simulink model "body_acc"  (R2019a)
settings: Solver=FixedStepAuto  StartTime=0.0  StopTime=inf  FixedStep=sT  RelTol=1e-3  EnableMultiTasking=on
InitFcn:
  | clear;
  | init_robot;
  | param;
values from neighbouring files (symbols this model uses):
  g = 9.80665    [param.m]    (also in sim_param.m)
  sT = 0.02    [param.m]    (also in sim_param.m = 0.001)
libraries: raspberrypilib x6, cstblocks x3
settings Model: SimulationMode=external  Creator=hideaki  LastModifiedBy=hideaki
settings SolverCC: PositivePriorityOrder=on
settings OptimizationCC: EnhancedBackFolding=on  PassReuseOutputArgsAs=Individual arguments  MaxStackSize=64  OptimizeBlockOrder=speed  DifferentSizesBufferReuse=on  OptimizationCustomize=off
settings DebuggingCC: ParameterTunabilityLossMsg=error  UnderSpecifiedDimensionMsg=warning
settings HardwareCC: ProdBitPerPointer=32  ProdBitPerSizeT=32  ProdBitPerPtrDiffT=32  ProdLargestAtomicInteger=Long  ProdLargestAtomicFloat=Double  ProdWordSize=32  ProdLongLongMode=on  ProdHWDeviceType=ARM Compatible->ARM Cortex  UseEmbeddedCoderFeatures=off  UseSimulinkCoderFeatures=off
settings SFSimCC: MATLABDynamicMemAlloc=off
settings RTWCC: SystemTargetFile=ert.tlc  HardwareBoard=Raspberry Pi  TLCOptions="-aInlineSetEventsForThisBaseRateFcn=TLC_FALSE -aSuppressMultiTaskScheduler=TLC_FALSE  -aRateBasedStepFcn=0"  TemplateMakefile=ert_default_tmf  RTWVerbose=off  Toolchain=GNU GCC Raspberry Pi  BuildConfiguration=Faster Runs  IncludeHyperlinkInReport=on
settings CodeAppCC: ForceParamTrailComments=on  OperatorAnnotations=on  SimulinkDataObjDesc=on  SFDataObjDesc=on  MangleLength=10  InsertBlockDesc=on
settings ERTTargetCC: SupportNonInlinedSFcns=on  SupportVariableSizeSignals=on  ExtMode=on  ExtModeMexArgs='192.168.10.103' 0 17725  ERTSrcFileBannerTemplate=codertarget_code_template.cgt  ERTHdrFileBannerTemplate=codertarget_code_template.cgt  ERTDataSrcFileTemplate=codertarget_code_template.cgt  ERTDataHdrFileTemplate=codertarget_code_template.cgt

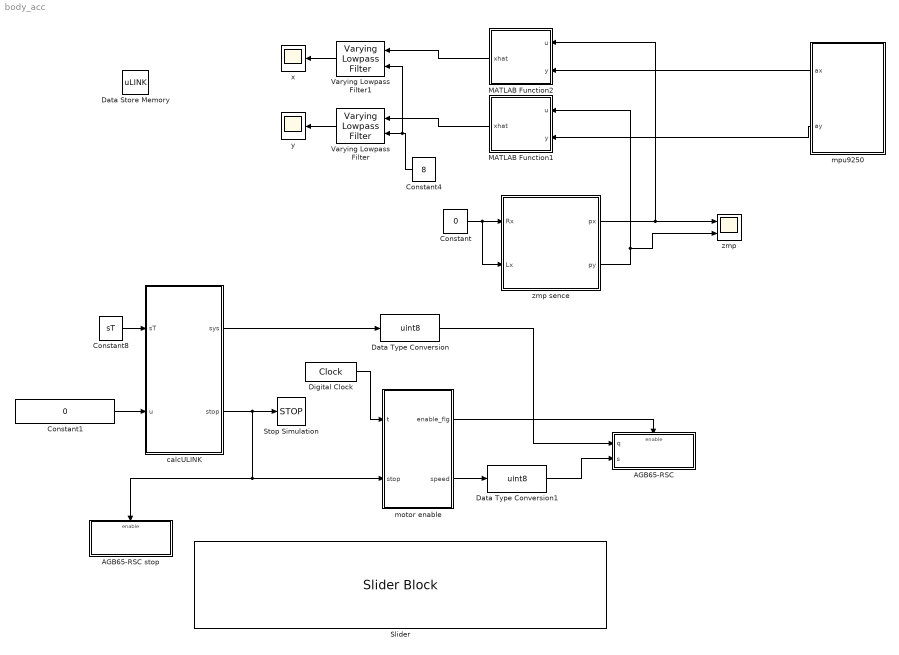
== system body_acc ==
  AGB65-RSC : Subsystem  TreatAsAtomicUnit=on
  AGB65-RSC stop : Subsystem  TreatAsAtomicUnit=on
  Constant : Constant  Value=0
  Constant1 : Constant  Value=0  OutDataTypeStr=double
  Constant4 : Constant  Value=8
  Constant8 : Constant  Value=sT
  Data Store Memory : DataStoreMemory  DataStoreName=uLINK  ReadBeforeWriteMsg=warning  WriteAfterWriteMsg=warning  WriteAfterReadMsg=warning  InitialValue=uLINK  ShowAdditionalParam=off  OutDataTypeStr=Bus: ULINK  Dimensions=[15 1]
  Data Type Conversion : DataTypeConversion  OutDataTypeStr=uint8
  Data Type Conversion1 : DataTypeConversion  OutDataTypeStr=uint8
  Digital Clock : DigitalClock  SampleTime=sT
  MATLAB Function1 : MATLAB Function  TreatAsAtomicUnit=on
  MATLAB Function2 : MATLAB Function  TreatAsAtomicUnit=on
  Slider : SliderBlock  LabelPosition=Hide  ScaleMin=-0.050000000000000003  ScaleMax=0.050000000000000003
  Stop Simulation : Stop
  Varying Lowpass Filter : cstblocks/Linear Parameter Varying/Varying Lowpass Filter  N=1
      settings: SourceProductName=Control System Toolbox
  Varying Lowpass Filter1 : cstblocks/Linear Parameter Varying/Varying Lowpass Filter  N=1
      settings: SourceProductName=Control System Toolbox
  calcULINK : MATLAB Function  TreatAsAtomicUnit=on
  motor enable : MATLAB Function  TreatAsAtomicUnit=on
  mpu9250 : Subsystem
  x : Scope
  y : Scope
  zmp : Scope  NumInputPorts=2
  zmp sence : Subsystem
  wires:
  Constant8/1 -> calcULINK/1(sT)
  Digital Clock/1 -> motor enable/1(t)
  Data Type Conversion1/1 -> AGB65-RSC/2(s)
  motor enable/1(enable_flg) -> AGB65-RSC/Enable
  Data Type Conversion/1 -> AGB65-RSC/1(q)
  calcULINK/1(sys) -> Data Type Conversion/1
  motor enable/2(speed) -> Data Type Conversion1/1
  calcULINK/2(stop) -> AGB65-RSC stop/Enable, motor enable/2(stop), Stop Simulation/1
  Constant/1 -> zmp sence/2(Lx), zmp sence/1(Rx)
  zmp sence/1(px) -> MATLAB Function2/1(u), zmp/1
  zmp sence/2(py) -> MATLAB Function1/1(u), zmp/2
  mpu9250/1(ax) -> MATLAB Function2/2(y)
  mpu9250/2(ay) -> MATLAB Function1/2(y)
  MATLAB Function1/1(xhat) -> Varying Lowpass Filter/1
  MATLAB Function2/1(xhat) -> Varying Lowpass Filter1/1
  Constant1/1 -> calcULINK/2(u)
  Constant4/1 -> Varying Lowpass Filter1/2, Varying Lowpass Filter/2
  Varying Lowpass Filter/1 -> y/1
  Varying Lowpass Filter1/1 -> x/1

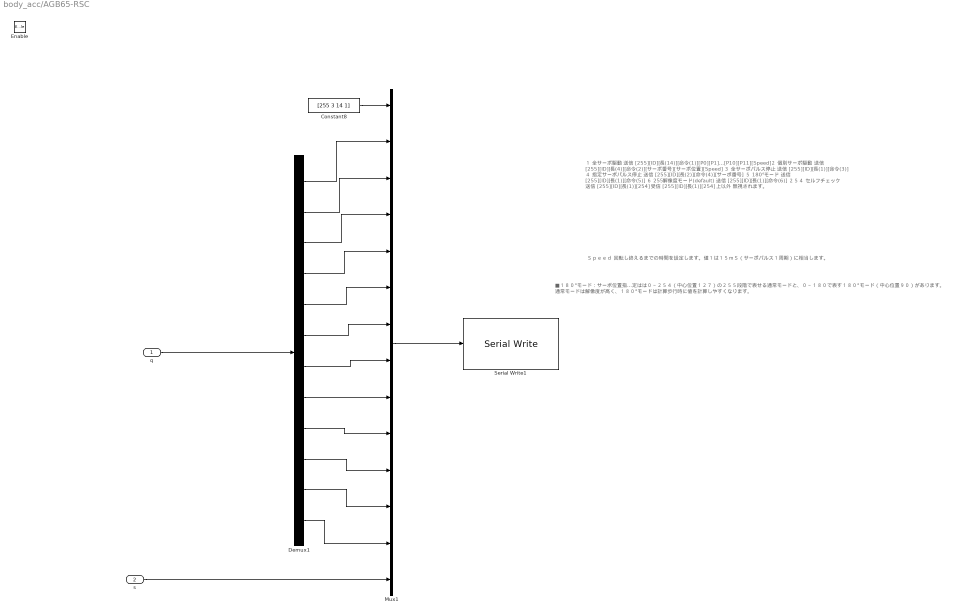
== system body_acc/AGB65-RSC ==
  note: Ｓｐｅｅｄ 回転し終えるまでの時間を設定します。値１は１５ｍＳ（サーボパルス１周期）に相当します。
  note: １ 全サーボ駆動 送信 [255][ID][長(14)][命令(1)][P0][P1]...[P10][P11][Speed]
      | ２ 個別サーボ駆動 送信 [255][ID][長(4)][命令(2)][サーボ番号][サーボ位置][Speed]
      | ３ 全サーボパルス停止 送信 [255][ID][長(1)][命令(3)]
      | ４ 指定サーボパルス停止 送信 [255][ID][長(2)][命令(4)][サーボ番号]
      | ５ 180°モード 送信 [255][ID][長(1)][命令(5)]
      | ６ 255解像度モード(default) 送信 [255][ID][長(1)][命令(6)]
      | ２５４ セルフチェック 送信 [255][ID][長(1)][254] 受信 [255][ID][長(1)][254]
      | 上以外 無視されます。
  note: ■１８０°モード：サーボ位置指定はは０～２５４（中心位置１２７）の２５５段階で表せる通常モードと、０～１８０で表す１８０°モード（中心位置９０）があります。
      | 通常モードは解像度が高く、１８０°モードは計算歩行時に値を計算しやすくなります。
  q : Inport
  s : Inport  Port=2
  Enable : EnablePort
  Constant8 : Constant  Value=[255 3 14 1]  OutDataTypeStr=uint8
  Demux1 : Demux  Outputs=12
  Mux1 : Mux  Inputs=14
  Serial Write1 : raspberrypilib/Serial Write  Priority=1  board=Pi 3 Model B  SCIModule_=/dev/ttyS0  Baudrate_=115200  Parity=None  StopBits_=1  HardwareFlowControl=None  ByteOrder=LittleEndian  OutputStatus=off  blockPlatform=RaspberryPi
      settings: SourceProductName=Simulink Support Package for Raspberry Pi Hardware  SourceProductBaseCode=RASPPI
  wires:
  Constant8/1 -> Mux1/1
  Demux1/11 -> Mux1/12
  q/1 -> Demux1/1
  Demux1/1 -> Mux1/2
  Demux1/3 -> Mux1/4
  Demux1/2 -> Mux1/3
  Mux1/1 -> Serial Write1/1
  Demux1/6 -> Mux1/7
  Demux1/10 -> Mux1/11
  Demux1/5 -> Mux1/6
  Demux1/7 -> Mux1/8
  Demux1/8 -> Mux1/9
  s/1 -> Mux1/14
  Demux1/9 -> Mux1/10
  Demux1/12 -> Mux1/13
  Demux1/4 -> Mux1/5

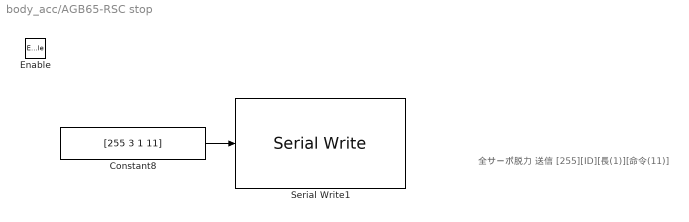
== system body_acc/AGB65-RSC stop ==
  note: 全サーボ脱力 送信 [255][ID][長(1)][命令(11)]
  Enable : EnablePort
  Constant8 : Constant  Value=[255 3 1 11]  OutDataTypeStr=uint8
  Serial Write1 : raspberrypilib/Serial Write  Priority=1  board=Pi 3 Model B  SCIModule_=/dev/ttyS0  Baudrate_=115200  Parity=None  StopBits_=1  HardwareFlowControl=None  ByteOrder=LittleEndian  OutputStatus=off  blockPlatform=RaspberryPi
      settings: SourceProductName=Simulink Support Package for Raspberry Pi Hardware  SourceProductBaseCode=RASPPI
  wires:
  Constant8/1 -> Serial Write1/1

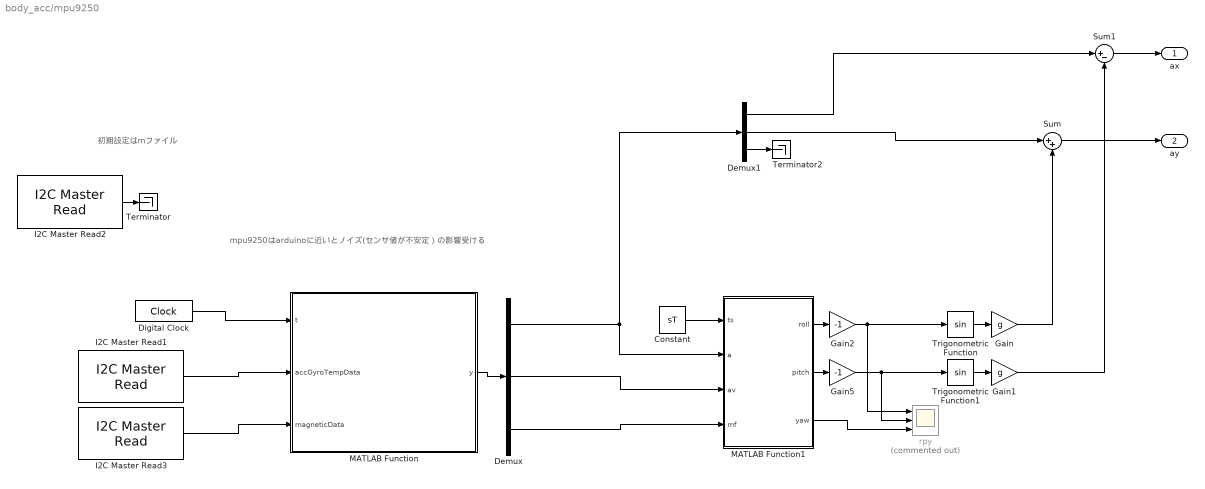
== system body_acc/mpu9250 ==
  note: mpu9250はarduinoに近いとノイズ(センサ値が不安定）の影響受ける
  note: 初期設定はmファイル
  Constant : Constant  Value=sT
  Demux : Demux  Outputs=3
  Demux1 : Demux  Outputs=3
  Digital Clock : DigitalClock  SampleTime=sT
  Gain : Gain  Gain=g
  Gain1 : Gain  Gain=g
  Gain2 : Gain  Gain=-1
  Gain5 : Gain  Gain=-1
  I2C Master Read1 : raspberrypilib/I2C Master Read  BoardProperty=Pi 3 Model B  Mode=Master  SlaveAddress=hex2dec( '68' )  SlaveByteOrder=BigEndian  Direction=Receiver  RegisterAddressMode=on  RegisterAddress=hex2dec( '3b' )  SlaveDataType=uint8  DataLength=14  NoAck=off  RepeatedStart=off  OutputStatus=off  SampleTime=-1
      settings: SourceProductName=Simulink Support Package for Raspberry Pi Hardware  SourceProductBaseCode=RASPPI
  I2C Master Read2 : raspberrypilib/I2C Master Read  BoardProperty=Pi 3 Model B  Mode=Master  SlaveAddress=hex2dec( '0c' )  SlaveByteOrder=BigEndian  Direction=Receiver  RegisterAddressMode=on  RegisterAddress=hex2dec( '02' )  SlaveDataType=uint8  DataLength=1  NoAck=off  RepeatedStart=off  OutputStatus=off  SampleTime=-1
      settings: SourceProductName=Simulink Support Package for Raspberry Pi Hardware  SourceProductBaseCode=RASPPI
  I2C Master Read3 : raspberrypilib/I2C Master Read  BoardProperty=Pi 3 Model B  Mode=Master  SlaveAddress=hex2dec( '0c' )  SlaveByteOrder=BigEndian  Direction=Receiver  RegisterAddressMode=on  RegisterAddress=hex2dec( '03' )  SlaveDataType=uint8  DataLength=7  NoAck=off  RepeatedStart=off  OutputStatus=off  SampleTime=-1
      settings: SourceProductName=Simulink Support Package for Raspberry Pi Hardware  SourceProductBaseCode=RASPPI
  MATLAB Function : MATLAB Function  TreatAsAtomicUnit=on
  MATLAB Function1 : MATLAB Function  TreatAsAtomicUnit=on
  Sum : Sum  Inputs=|++
  Sum1 : Sum  Inputs=|+-
  Terminator : Terminator
  Terminator2 : Terminator
  Trigonometric Function : Trigonometry
  Trigonometric Function1 : Trigonometry
  rpy : Scope  Commented=on  NumInputPorts=3
  ax : Outport
  ay : Outport  Port=2
  wires:
  I2C Master Read2/1 -> Terminator/1
  Constant/1 -> MATLAB Function1/1(ts)
  I2C Master Read3/1 -> MATLAB Function/3(magneticData)
  Demux/2 -> MATLAB Function1/3(av)
  Sum/1 -> ay/1
  Demux/1 -> Demux1/1, MATLAB Function1/2(a)
  Demux/3 -> MATLAB Function1/4(mf)
  Gain/1 -> Sum/2
  I2C Master Read1/1 -> MATLAB Function/2(accGyroTempData)
  Trigonometric Function/1 -> Gain/1
  Sum1/1 -> ax/1
  Trigonometric Function1/1 -> Gain1/1
  MATLAB Function1/2(pitch) -> Gain5/1
  Gain1/1 -> Sum1/2
  MATLAB Function1/1(roll) -> Gain2/1
  Demux1/1 -> Sum1/1
  Digital Clock/1 -> MATLAB Function/1(t)
  MATLAB Function/1(y) -> Demux/1
  MATLAB Function1/3(yaw) -> rpy/3
  Demux1/3 -> Terminator2/1
  Demux1/2 -> Sum/1
  Gain5/1 -> rpy/2, Trigonometric Function1/1
  Gain2/1 -> rpy/1, Trigonometric Function/1

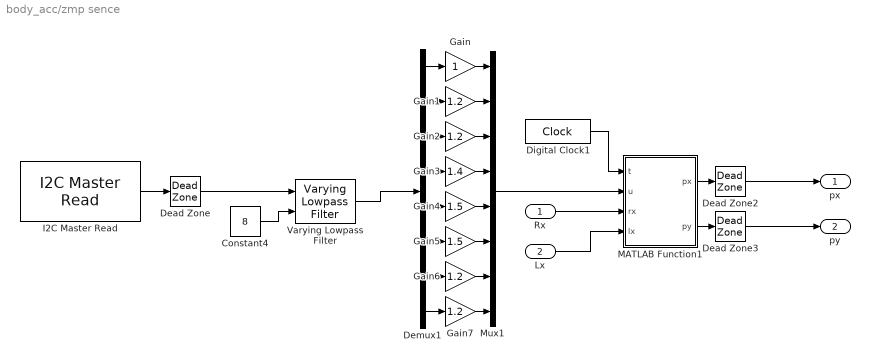
== system body_acc/zmp sence ==
  Rx : Inport
  Lx : Inport  Port=2
  Constant4 : Constant  Value=8
  Dead Zone : DeadZone  LowerValue=0  UpperValue=5  SaturateOnIntegerOverflow=on
  Dead Zone2 : DeadZone  LowerValue=-1e-5  UpperValue=1e-5  SaturateOnIntegerOverflow=on
  Dead Zone3 : DeadZone  LowerValue=-1e-5  UpperValue=1e-5  SaturateOnIntegerOverflow=on
  Demux1 : Demux  Outputs=8
  Digital Clock1 : DigitalClock  SampleTime=sT
  Gain : Gain
  Gain{1..2,6..7} (4 alike) : Gain  Gain=1.2
  Gain3 : Gain  Gain=1.4
  Gain4 : Gain  Gain=1.5
  Gain5 : Gain  Gain=1.5
  I2C Master Read : raspberrypilib/I2C Master Read  BoardProperty=Pi 3 Model B  Mode=Master  SlaveAddress=hex2dec( '04' )  SlaveByteOrder=BigEndian  Direction=Receiver  RegisterAddressMode=off  RegisterAddress=hex2dec( '20' )  SlaveDataType=uint8  DataLength=8  NoAck=off  RepeatedStart=off  OutputStatus=off  SampleTime=sT
      settings: SourceProductName=Simulink Support Package for Raspberry Pi Hardware  SourceProductBaseCode=RASPPI
  MATLAB Function1 : MATLAB Function  TreatAsAtomicUnit=on
  Mux1 : Mux  Inputs=8
  Varying Lowpass Filter : cstblocks/Linear Parameter Varying/Varying Lowpass Filter  N=1
      settings: SourceProductName=Control System Toolbox
  px : Outport
  py : Outport  Port=2
  wires:
  Mux1/1 -> MATLAB Function1/2(u)
  Demux1/5 -> Gain4/1
  Demux1/6 -> Gain5/1
  Varying Lowpass Filter/1 -> Demux1/1
  Constant4/1 -> Varying Lowpass Filter/2
  I2C Master Read/1 -> Dead Zone/1
  Demux1/1 -> Gain/1
  Gain/1 -> Mux1/1
  Gain2/1 -> Mux1/3
  Gain4/1 -> Mux1/5
  Gain1/1 -> Mux1/2
  MATLAB Function1/1(px) -> Dead Zone2/1
  Gain3/1 -> Mux1/4
  Gain6/1 -> Mux1/7
  Gain7/1 -> Mux1/8
  Dead Zone/1 -> Varying Lowpass Filter/1
  Demux1/3 -> Gain2/1
  Demux1/7 -> Gain6/1
  Demux1/2 -> Gain1/1
  Digital Clock1/1 -> MATLAB Function1/1(t)
  Demux1/8 -> Gain7/1
  Gain5/1 -> Mux1/6
  Demux1/4 -> Gain3/1
  MATLAB Function1/2(py) -> Dead Zone3/1
  Dead Zone2/1 -> px/1
  Rx/1 -> MATLAB Function1/3(rx)
  Lx/1 -> MATLAB Function1/4(lx)
  Dead Zone3/1 -> py/1

== matlab function body_acc/motor enable ==
  data: t input; enable_flg output; speed output; stop input
function [enable_flg,speed]= fcn(t,stop)
    
    enable_flg = 0;
    speed = 1;
    persistent cnt;
    if isempty(cnt)
        cnt = 0;
    end
    
    if (stop == 1) 
        enable_flg = 0;
    else
        if (cnt == 0)
            enable_flg = 1;
            speed = 30;
            cnt = cnt+1;
        elseif (t <= 5)
            enable_flg = 0;
        else
            enable_flg = 1;
        end
    end
end

== matlab function body_acc/MATLAB Function2 ==
  settings: updateMethod=DISCRETE
  data: u input; y input; xhat output
function xhat = kf(u,y)
    
    persistent x;
    if isempty(x)
        x = zeros(2, 1);
    end
    persistent P;
    if isempty(P)
        P = 0.1*eye(2);
    end
    
    Ad = [1.0073 0.0200;
        0.7282 1.0073];
    Bd = [-0.0073;
        -0.7282];
    Cd = [36.3209 0];
    Dd = -36.3209;
    
    %%共分散行列
    %Qを大きくするとzmpに近い出力
    Q = 0;
    R = 1;
    
    I = eye(2);
    %%カルマンフィルタ
    x = Ad*x+Bd*u;
    P = Ad*P*Ad'+Q;
    K = (P*Cd')/(Cd*P*Cd'+R);
    x = x+K*(y-Cd*x-Dd*u);
    P = (I-K*Cd)*P;

    xhat = x;
    
end

== matlab function body_acc/mpu9250/MATLAB Function ==
  settings: updateMethod=DISCRETE
  data: t input; accGyroTempData input; y output; magneticData input
function y = out_mpu9250(t,accGyroTempData,magneticData)

    y = zeros(9,1);
    
    %計算で使用するので，選択したレンジを入力する
    accRange = 16.0;
    %%計算で使用するので，選択したレンジを入力する
    gyroRange = 2000.0;
    
    %%Acc
    ax = -nbin2dec(dec2bin(bitshift(uint16(accGyroTempData(1)),8) + uint16(accGyroTempData(2)),16));
    ay = nbin2dec(dec2bin(bitshift(uint16(accGyroTempData(3)),8) + uint16(accGyroTempData(4)),16));
    az = nbin2dec(dec2bin(bitshift(uint16(accGyroTempData(5)),8) + uint16(accGyroTempData(6)),16));
    
    %%Gyro
    gx = nbin2dec(dec2bin(bitshift(uint16(accGyroTempData(9)),8) + uint16(accGyroTempData(10)),16));
    gy = nbin2dec(dec2bin(bitshift(uint16(accGyroTempData(11)),8) + uint16(accGyroTempData(12)),16));
    gz = nbin2dec(dec2bin(bitshift(uint16(accGyroTempData(13)),8) + uint16(accGyroTempData(14)),16));
    
    %%Temp
    %tempMPU9250Raw = bitshift(accGyroTempData(7),8) | accGyroTempData(8);%accGyroTempData[6]を左に8シフトし(<<)，accGyroTempData[7]を足し合わせる(|)
    
    %%Magneto
    mx = nbin2dec(dec2bin(bitshift(uint16(magneticData(4)),8) + uint16(magneticData(3)),16));
    my = nbin2dec(dec2bin(bitshift(uint16(magneticData(2)),8) + uint16(magneticData(1)),16));
    mz = -(nbin2dec(dec2bin(bitshift(uint16(magneticData(6)),8) + uint16(magneticData(5)),16)));
    
    %加速度
    %16bit(最大値32768)を16Gで割る
    ax = ax * accRange / 32768.0;%[G]に変換
    ay = ay * accRange / 32768.0;%[G]に変換
    az = az * accRange / 32768.0;%[G]に変換
    
    %角加速度
    gx = gx * gyroRange / 32768.0;%[deg/s]に変換
    gy = gy * gyroRange / 32768.0;%[deg/s]に変換
    gz = gz * gyroRange / 32768.0;%[deg/s]に変換
    
    persistent idx; 
    if isempty(idx) 
        idx = 1; 
    end
    
    %最初の100までの平均値
    persistent ax_100;
    persistent ay_100;
    %persistent az_100;
    persistent ax_avg;
    persistent ay_avg;
    %persistent az_avg;
    
    persistent gx_100;
    persistent gy_100;
    persistent gz_100;
    persistent gx_avg;
    persistent gy_avg;
    persistent gz_avg;
    if isempty(gx_100)
        ax_100 = zeros(1, 100);
        ay_100 = zeros(1, 100);
        %az_100 = zeros(1, 100);
        ax_avg = 0;
        ay_avg = 0;
        %az_avg = 0;
        
        gx_100 = zeros(1, 100);
        gy_100 = zeros(1, 100);
        gz_100 = zeros(1, 100);
        gx_avg = 0;
        gy_avg = 0;
        gz_avg = 0;
    end
    
    y = zeros(9,1);
    if (t < 2)
        
    elseif (t >= 2 && idx <= 100)
        ax_100(idx) = ax;
        ay_100(idx) = ay;
        %az_100(idx) = az;
        ax_avg = mean(ax_100);
        ay_avg = mean(ay_100);
        %az_avg = mean(az_100);
        
        gx_100(idx) = gx;
        gy_100(idx) = gy;
        gz_100(idx) = gz;
        gx_avg = mean(gx_100);
        gy_avg = mean(gy_100);
        gz_avg = mean(gz_100);
        
        idx = idx+1;
        
    else
        
        ax = ax-ax_avg;
        ay = ay-ay_avg;
        %az = az-az_avg;
        
        gx = gx-gx_avg;
        gy = gy-gy_avg;
        gz = gz-gz_avg;
        
        %[G]→[m/s^2]
        y(1) = ax*9.80665;
        y(2) = ay*9.80665;
        y(3) = az*9.80665;

        y(4) = deg2rad(gx);
        y(5) = deg2rad(gy);
        y(6) = deg2rad(gz);

        %tempMPU9250 = ((tempMPU9250Raw - 0.0) / 333.87) + 21.0;

        %方位
        mx = mx / 32768.0 * 4800.0;%[uT]に変換
        my = my / 32768.0 * 4800.0;%[uT]に変換
        mz = mz / 32768.0 * 4800.0;%[uT]に変換

        %感度とオフセット
        Gx = 1;
        bx = 27.4;
        Gy = 0.9;
        by = 9;
        Gz = 1;
        bz = 30;

        %パラメータ補正
        mfx = (mx-bx)/Gx;
        mfy = (my-by)/Gy;
        mfz = (mz-bz)/Gz;

        y(7) = mfx;
        y(8) = mfy;
        y(9) = mfz;
    end
    
    
end

== matlab function body_acc/mpu9250/MATLAB Function1 ==
  settings: updateMethod=DISCRETE
  data: ts input; a input; av input; roll output; mf input; pitch output; yaw output
function [roll, pitch, yaw] = kf(ts, a, av, mf)
    
    persistent cnt;
    if isempty(cnt)
        cnt = 0;
    end
    if (cnt < 102)
        cnt = cnt+1;
    end
    
    persistent x;
    if isempty(x)
        x = zeros(3, 1);
    end
    persistent P;
    if isempty(P)
        P = 0.1*eye(3);
    end
    
    persistent yawm_100;
    persistent yawm_avg;
    if isempty(yawm_100)
        yawm_100 = zeros(1, 100);
        yawm_avg = 0;
    end
    
    roll = 0;
    pitch = 0;
    yaw = 0;
        
    rolla = atan2(a(2), a(3));
    pitcha = atan2(-a(1), sqrt(a(2)*a(2)+a(3)*a(3)));
    
    if (cnt <= 100)
        
        %傾斜誤差補正
        M = [cos(pitcha) sin(rolla)*sin(pitcha) cos(rolla)*sin(pitcha);
            0 cos(rolla) -sin(rolla);
            -sin(pitcha) sin(rolla)*cos(pitcha) cos(rolla)*cos(pitcha)];
        m = M*[mf(1);mf(2);mf(3)];

        %yaw
        yawm = atan2(-m(2), m(1));
        yawm_100(cnt) = yawm;
        yawm_avg = mean(yawm_100(cnt));
        
        x(1) = yawm;
        x(2) = pitcha;
        x(3) = rolla;
        
        roll = rolla;
        pitch = pitcha;
        yaw = yawm-yawm_avg;
        %yaw = yawm;
        
    else
        
        I = eye(3);
        
        %%共分散行列
        Q = [160 0 0;
            0 160 0;
            0 0 160];
        R = [20 0 0;
            0 20 0;
            0 0 20];
        
        B = [0 sin(x(3))/cos(x(2)) cos(x(3))/cos(x(2));
            0 cos(x(3)) -sin(x(3));
            1 sin(x(3))*tan(x(2)) cos(x(3))*tan(x(2))];
        
        u = [av(1)*ts;av(2)*ts;av(3)*ts];
        
        %%傾斜誤差補正
        M = [cos(x(2)) sin(x(3))*sin(x(2)) cos(x(3))*sin(x(2));
            0 cos(x(3)) -sin(x(3));
            -sin(x(2)) sin(x(3))*cos(x(2)) cos(x(3))*cos(x(2))];
        m = M*[mf(1);mf(2);mf(3)];

        yawm = atan2(-m(2), m(1))-yawm_avg;
        %yawm = atan2(-m(2), m(1));
        
        y = [yawm;pitcha;rolla];
        
        %%カルマンフィルタ
        x = I*x+B*u;
        P = I*P*I'+Q;
        K = (P*I')/(I*P*I'+R);
        x = x+K*(y-I*x);
        P = (I-K*I)*P;
        
        roll = x(3);
        pitch = x(2);
        yaw = x(1);
        
    end
    
end

== matlab function body_acc/calcULINK ==
  settings: updateMethod=DISCRETE
  data: sT input; u input; sys output; uLINK data_store_memory; stop output
function [sys,stop] = calcULINK(sT,u)

    %u[腰X 腰Y 右足X 右足Y 右足Z 左足X 左足Y 左足Z]
    
    stop = 0;
    global uLINK;
    
    persistent cnt;
    if isempty(cnt)
        cnt = 0.0;
    end
    
    ToDeg = 180/pi;
    ToRad = pi/180;
    
    sys = zeros(12,1);
    
    %%% ZMPの計算
    %com = calcCoM;  % 重心位置
    %P = calcP(1);   % 並進運動量
    %L = calcL(1);   % 原点回りの角運動量
    
    %Zc  = com(3);      % 線形倒立振子の設定高さ
    %Tc  = sqrt(Zc/G);  % 線形倒立振子の時定数
    %cx0 = com(1);
    %cy0 = com(2);
    
    p0 = uLINK(JointName.BODY).p;
    uLINK(JointName.BODY).p = [0, u, uLINK(JointName.BODY).p(3)]';
    v = (uLINK(JointName.BODY).p-p0)/sT;
    uLINK(JointName.BODY).v = [v(1) v(2) v(3)]';
    uLINK(JointName.BODY).R = RPY2R([0 0*ToRad 0]);

    %ForwardKinematics(1);
    
    p = [0 -0.04 0]';
    Rfoot.p = p;
    Rfoot.R = RPY2R([0 0 0]);
    v = (p-uLINK(JointName.RLEG_FOOT).p)/sT;
    Rfoot.v = [v(1) v(2) v(3)]';
    Rfoot.w = [0 0 0]';
    InverseKinematicsAll(8, Rfoot);
    
    p = [0 0.04 0]';
    Lfoot.p = p;
    Lfoot.R = RPY2R([0 0 0]);
    v = (p-uLINK(JointName.LLEG_FOOT).p)/sT;
    Lfoot.v = [v(1) v(2) v(3)]';
    Lfoot.w = [0 0 0]';
    InverseKinematicsAll(15, Lfoot);
    
    ForwardVelocity(1); 
    
    %{
    p0 = uLINK(JointName.BODY).p;
    uLINK(JointName.BODY).p = [u(1), u(2), uLINK(JointName.BODY).p(3)]';
    v = (uLINK(JointName.BODY).p-p0)/sT;
    uLINK(JointName.BODY).v = [v(1) v(2) v(3)]';
    uLINK(JointName.BODY).R = RPY2R([0 0*ToRad 0]);

    %ForwardKinematics(1);
    
    p = [u(3) u(4) u(5)]';
    Rfoot.p = [u(3) u(4) u(5)]';
    Rfoot.R = RPY2R([0 0 0]);
    v = (p-uLINK(JointName.RLEG_FOOT).p)/sT;
    Rfoot.v = [v(1) v(2) v(3)]';
    Rfoot.w = [0 0 0]';
    InverseKinematicsAll(8, Rfoot);
    
    p = [u(6) u(7) u(8)]';
    Lfoot.p = [u(6) u(7) u(8)]';
    Lfoot.R = RPY2R([0 0 0]);
    v = (p-uLINK(JointName.LLEG_FOOT).p)/sT;
    Lfoot.v = [v(1) v(2) v(3)]';
    Lfoot.w = [0 0 0]';
    InverseKinematicsAll(15, Lfoot);
    
    ForwardVelocity(1); 
    %}
    
    
    sys = [90 90 90 90 90 90 90 90 90 90 90 90]';
    
    if (abs(rad2deg(uLINK(JointName.RLEG_J0).q)) > 30 || abs(rad2deg(uLINK(JointName.LLEG_J0).q)) > 30)
        stop = 1;
    end
    if (abs(rad2deg(uLINK(JointName.RLEG_J1).q)) > 60 || abs(rad2deg(uLINK(JointName.LLEG_J1).q)) > 60 || ...
        abs(rad2deg(uLINK(JointName.RLEG_J5).q)) > 60 || abs(rad2deg(uLINK(JointName.LLEG_J5).q)) > 60)
        stop = 1;
    end
    if (abs(rad2deg(uLINK(JointName.RLEG_J2).q)) > 60 || abs(rad2deg(uLINK(JointName.LLEG_J2).q)) > 60 || ...
        abs(rad2deg(uLINK(JointName.RLEG_J4).q)) > 60 || abs(rad2deg(uLINK(JointName.LLEG_J4).q)) > 60)
        stop = 1;
    end
    if (abs(rad2deg(uLINK(JointName.RLEG_J3).q)) > 90 || abs(rad2deg(uLINK(JointName.LLEG_J3).q)) > 90)
        stop = 1;
    end
    
    sys(1) = round(rad2deg(uLINK(JointName.RLEG_J0).q))+90;
    %股関節の剛性不足による胴体の傾き補償フィードフォワード
    sys(2) = round(rad2deg(uLINK(JointName.RLEG_J1).q))+90-1;
    sys(3) = -round(rad2deg(uLINK(JointName.RLEG_J2).q))+90;
    sys(4) = -round(rad2deg(uLINK(JointName.RLEG_J3).q))+90;
    sys(5) = -round(rad2deg(uLINK(JointName.RLEG_J4).q))+90;
    sys(6) = -round(rad2deg(uLINK(JointName.RLEG_J5).q))+90;
    
    sys(7) = round(rad2deg(uLINK(JointName.LLEG_J0).q))+90;
    sys(8) = round(rad2deg(uLINK(JointName.LLEG_J1).q))+90+1;
    sys(9) = -round(rad2deg(uLINK(JointName.LLEG_J2).q))+90;
    sys(10) = -round(rad2deg(uLINK(JointName.LLEG_J3).q))+90;
    sys(11) = -round(rad2deg(uLINK(JointName.LLEG_J4).q))+90;
    sys(12) = -round(rad2deg(uLINK(JointName.LLEG_J5).q))+90;
    
    for i = 1:12
        if (abs(sys(i)) > 180)
            stop = 1;
        end
    end
   
    
    cnt = cnt + sT;
end

== matlab function body_acc/zmp sence/MATLAB Function1 ==
  settings: updateMethod=DISCRETE
  data: t input; u input; px output; py output; rx input; lx input
function [px,py] = fcn(t,u,rx,lx)
    
    r = -0.04;
    l = 0.04;
    xs = 0.07/2;
    ys = 0.045/2;
    
    
    r1x = (rx+xs)*u(1);
    r2x = (rx+xs)*u(2);
    r3x = (rx-xs)*u(3);
    r4x = (rx-xs)*u(4);
    PrxfRz = r1x+r2x+r3x+r4x;
    
    r1y = (r+ys)*u(1);
    r2y = (r-ys)*u(2);
    r3y = (r+ys)*u(3);
    r4y = (r-ys)*u(4);
    PryfRz = r1y+r2y+r3y+r4y;
    
    l1x = (lx+xs)*u(5);
    l2x = (lx+xs)*u(6);
    l3x = (lx-xs)*u(7);
    l4x = (lx-xs)*u(8);
    PlxfLz = l1x+l2x+l3x+l4x;
    
    l1y = (l+ys)*u(5);
    l2y = (l-ys)*u(6);
    l3y = (l+ys)*u(7);
    l4y = (l-ys)*u(8);
    PlyfLz = l1y+l2y+l3y+l4y;
    
    fRz = u(1)+u(2)+u(3)+u(4);
    fLz = u(5)+u(6)+u(7)+u(8);
    
    %両足が浮いてない
    if (fRz+fLz ~= 0 && t > 5) 
        %x軸のずれ0.02加算
        px = (PrxfRz+PlxfLz)/(fRz+fLz)+0.003;
        py = (PryfRz+PlyfLz)/(fRz+fLz)+0.005;
    else
        px = 0;
        py = 0;
    end
    
    %{
    FnR_FrontLeft
    FnR_FrontRight
    FnR_RearLeft
    FnR_RearRight
    
    
    FnL_FrontLeft
    FnL_FrontRight
    FnL_RearLeft
    FnL_RearRight
    %}
    
    
end

== matlab function body_acc/MATLAB Function1 ==
  settings: updateMethod=DISCRETE
  data: u input; y input; xhat output
function xhat = kf(u,y)
    
    persistent x;
    if isempty(x)
        x = zeros(2, 1);
    end
    persistent P;
    if isempty(P)
        P = 0.1*eye(2);
    end
    
    Ad = [1.0073 0.0200;
        0.7282 1.0073];
    Bd = [-0.0073;
        -0.7282];
    Cd = [36.3209 0];
    Dd = -36.3209;
    
    %%共分散行列
    %Qを大きくするとzmpに近い出力
    Q = 0;
    R = 1;
    
    I = eye(2);
    %%カルマンフィルタ
    x = Ad*x+Bd*u;
    P = Ad*P*Ad'+Q;
    K = (P*Cd')/(Cd*P*Cd'+R);
    x = x+K*(y-Cd*x-Dd*u);
    P = (I-K*Cd)*P;

    xhat = x;
    
end
